simulink model "DA40_Flight_Model"  (R2023a)
settings: Solver=FixedStepAuto  StartTime=Start_Time  StopTime=End_Time  FixedStep=Time_Step  RelTol=1e-3
values from neighbouring files (symbols this model uses):
  BSFC_LUT = aircraft.BSFC_LUT    [NavigationProcessor.m]    (also in ReceiverPositions.m = obj.aircraft.BSFC_LUT; VectorTracking.m = load("DA40ENGINE.mat"))
  clkVar = formClkVariance(aircraft.clockType,1/aircraft.frequency)    [initializeSim.m]
  initP = blkdiag(diag([0.1 0.1 0.1]),diag([pi/90 pi/90 pi/90]),diag([1 1 1]),diag([pi/45 pi/45 pi/45]),clkVar)    [initializeSim.m]
  Q = blkdiag(diag(str2num(cell2mat(aircraft.noiseVariance))),clkVar)    [initializeSim.m]
  STGeometry = aircraft.STGeometry    [NavigationProcessor.m]    (also in ReceiverPositions.m = obj.aircraft.STGeometry; VectorTracking.m = load("DA40STGEOM.mat"))
  Vehicle = aircraft.Vehicle    [NavigationProcessor.m]    (also in ReceiverPositions.m = obj.aircraft.Vehicle; VectorTracking.m = load("DA40.mat"))
undefined symbols (not defined in the file or in its folder): day, initCN0, Initial_X, month, PowerFactor_LUT, Time_Step, unifrnd, variance, year
libraries: slpidlib x8, simulink_extras x3, aerolibwind2 x2, aerolibatmos2 x2, simulink x1
(part 2 of 2)

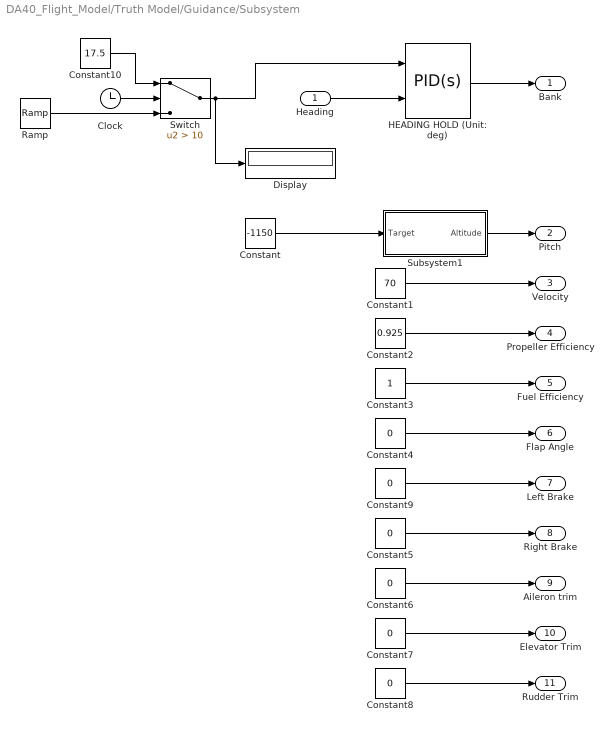
== system DA40_Flight_Model/Truth Model/Guidance/Subsystem ==
  Heading : Inport
  Clock : Clock
  Constant : Constant  Value=-1150
  Constant1 : Constant  Value=70
  Constant10 : Constant  Value=17.5
  Constant2 : Constant  Value=0.925
  Constant3 : Constant
  Constant{4..9} (6 alike) : Constant  Value=0
  Display : Display
  HEADING HOLD (Unit: deg) : slpidlib/PID Controller (2DOF)  Controller=PID  Form=Parallel  TimeDomain=Continuous-time  UseExternalTs=off  SampleTime=-1  IntegratorMethod=Forward Euler  FilterMethod=Forward Euler  ControllerParametersSource=internal  P=1  I=0.001  UseKiTs=off  D=0  N=100  UseFilter=on  b=1  c=0  TunerSelectOption=Transfer Function Based (PID Tuner App)  InitialConditionSource=internal  InitialConditionForIntegrator=0  InitialConditionForFilter=0  DifferentiatorICPrevScaledInput=0  ExternalReset=none  TrackingMode=off  Kt=1  LimitOutput=on  SatLimitsSource=internal  UpperSaturationLimit=30  LowerSaturationLimit=-30  LinearizeAsGain=on  AntiWindupMode=clamping  Kb=1  LimitIntegrator=off  UpperIntegratorSaturationLimit=inf  LowerIntegratorSaturationLimit=-inf  POutMin=[]  POutMax=[]  IOutMin=[]  IOutMax=[]  DOutMin=[]  DOutMax=[]  NOutMin=[]  NOutMax=[]  bOutMin=[]  bOutMax=[]  cOutMin=[]  cOutMax=[]  SumOutMin=[]  SumOutMax=[]  SaturationOutMin=[]  SaturationOutMax=[]  PParamMin=[]  PParamMax=[]  IParamMin=[]  IParamMax=[]  DParamMin=[]  DParamMax=[]  NParamMin=[]  NParamMax=[]  bParamMin=[]  bParamMax=[]  cParamMin=[]  cParamMax=[]  KbParamMin=[]  KbParamMax=[]  KtParamMin=[]  KtParamMax=[]  KbOutMin=[]  KbOutMax=[]  KtOutMin=[]  KtOutMax=[]  IntegratorOutMin=[]  IntegratorOutMax=[]  FilterOutMin=[]  FilterOutMax=[]  SumI1OutMin=[]  SumI1OutMax=[]  SumI2OutMin=[]  SumI2OutMax=[]  SumI3OutMin=[]  SumI3OutMax=[]  SumI4OutMin=[]  SumI4OutMax=[]  SumDOutMin=[]  SumDOutMax=[]  Sum1OutMin=[]  Sum1OutMax=[]  Sum2OutMin=[]  Sum2OutMax=[]  Sum3OutMin=[]  Sum3OutMax=[]  DifferentiatorOutMin=[]  DifferentiatorOutMax=[]  FilterDiffOutCoefMin=[]  FilterDiffOutCoefMax=[]  ReciprocalOutMin=[]  ReciprocalOutMax=[]  SumDenOutMin=[]  SumDenOutMax=[]  SumNumOutMin=[]  SumNumOutMax=[]  DivideOutMin=[]  DivideOutMax=[]  UdiffTsProdOutMin=[]  UdiffTsProdOutMax=[]  NTsProdOutMin=[]  NTsProdOutMax=[]  UintegralTsProdOutMin=[]  UintegralTsProdOutMax=[]  UngainTsProdOutMin=[]  UngainTsProdOutMax=[]  ClampingZeroOutDataTypeStr=Inherit: Inherit via back propagation  ClampingZeroOutMin=[]  ClampingZeroOutMax=[]  FilterDenConstantOutDataTypeStr=Inherit: Inherit via back propagation  FilterDenConstantOutMin=[]  FilterDenConstantOutMax=[]  PCopyOutDataTypeStr=Inherit: Inherit via back propagation  PCopyOutMin=[]  PCopyOutMax=[]  NCopyOutDataTypeStr=Inherit: Inherit via back propagation  NCopyOutMin=[]  NCopyOutMax=[]  IntegratorContinuousStateAttributes=''  IntegratorStateMustResolveToSignalObject=off  IntegratorRTWStateStorageClass=Auto  FilterContinuousStateAttributes=''  FilterStateMustResolveToSignalObject=off  FilterRTWStateStorageClass=Auto  ParallelPVariant=InternalParameters  IdealPVariant=Disabled  IVariant=InternalParameters  DVariant=InternalParameters  bVariant=InternalParameters  cVariant=InternalParameters  IntegratorVariant=Continuous  SatVariant=Enabled  AWVariant=ContClampingParallel  PCopyVariant=Disabled  TRVariant=Disabled  FdbkBlocksVariant=Forward  IdealPFdbkVariant=Disabled  SatFdbkVariant=Disabled  DerivativeFilterVariant=ContFilter  NVariant=InternalParameters  NCopyVariant=Disabled  FilterICVariant=InternalICsFilter  IntegratorICVariant=InternalICs  ExternalResetVariant=Disabled  TRSumVariant=Passthrough  SumFdbkVariant=Disabled  SumVariant=Sum_PID  TsampFilterVariant=InternalTs  TsampNgainVariant=Passthrough  TsampIntegralVariant=Disabled_SignalSpec  ExternalSaturationOutDataTypeStr=Inherit: Same as second input
  Ramp : simulink/Sources/Ramp  slope=2  start=1  InitialOutput=0  VectorParams1D=off
  Subsystem1 : Subsystem
  Switch : Switch  Criteria=u2 > Threshold  Threshold=10  SaturateOnIntegerOverflow=off  InputSameDT=off
  Bank : Outport
  Pitch : Outport  Port=2
  Velocity : Outport  Port=3
  Propeller Efficiency : Outport  Port=4
  Fuel Efficiency : Outport  Port=5
  Flap Angle : Outport  Port=6
  Left Brake : Outport  Port=7
  Right Brake : Outport  Port=8
  Aileron trim : Outport  Port=9
  Elevator Trim : Outport  Port=10
  Rudder Trim : Outport  Port=11
  wires:
  Subsystem1/1(Altitude) -> Pitch/1
  Constant1/1 -> Velocity/1
  Constant2/1 -> Propeller Efficiency/1
  Constant3/1 -> Fuel Efficiency/1
  Constant4/1 -> Flap Angle/1
  Constant9/1 -> Left Brake/1
  Constant5/1 -> Right Brake/1
  Constant6/1 -> Aileron trim/1
  Constant7/1 -> Elevator Trim/1
  Constant8/1 -> Rudder Trim/1
  HEADING HOLD (Unit: deg)/1 -> Bank/1
  Heading/1 -> HEADING HOLD (Unit: deg)/2
  Constant/1 -> Subsystem1/1(Target)
  Clock/1 -> Switch/2
  Ramp/1 -> Switch/3
  Constant10/1 -> Switch/1
  Switch/1 -> Display/1, HEADING HOLD (Unit: deg)/1

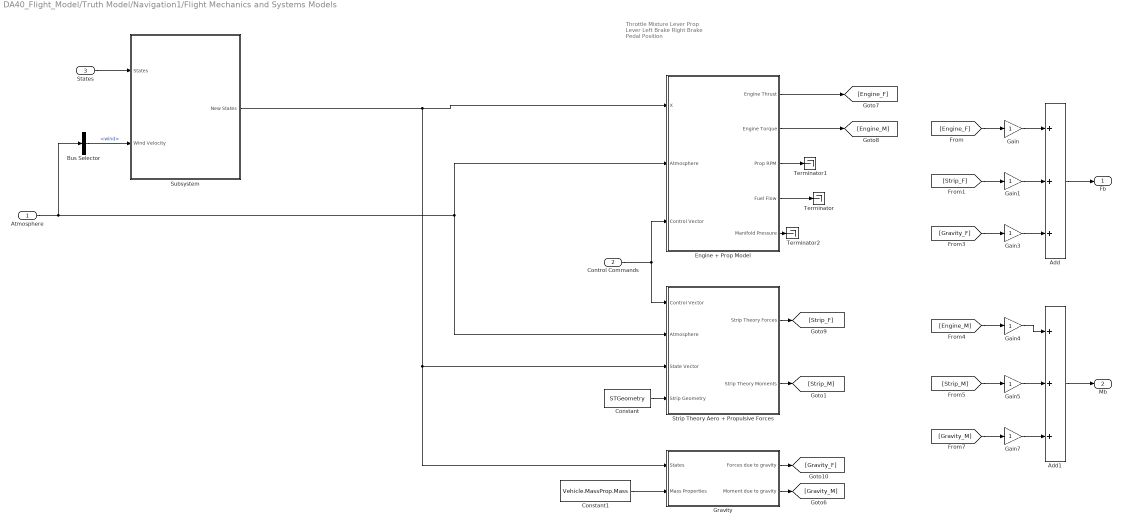
== system DA40_Flight_Model/Truth Model/Navigation1/Flight Mechanics and Systems Models ==
  note: Throttle
      | Mixture Lever
      | Prop Lever
      | Left Brake
      | Right Brake
      | Pedal Position
  Atmosphere : Inport
  Control Commands : Inport  Port=2
  States : Inport  Port=3
  Add : Sum  Inputs=+++
  Add1 : Sum  Inputs=+++
  Bus Selector : BusSelector  OutputSignals=wind
  Constant : Constant  Value=STGeometry
  Constant1 : Constant  Value=Vehicle.MassProp.Mass
  Engine + Prop Model : Subsystem
  Gain{,1,3..5,7} (6 alike) : Gain
  Gravity : Subsystem
  Strip Theory Aero + Propulsive Forces : Subsystem
  Subsystem : Subsystem
  Terminator : Terminator
  Terminator1 : Terminator
  Terminator2 : Terminator
  Fb : Outport
  Mb : Outport  Port=2
  wires:
  Constant1/1 -> Gravity/2(Mass Properties)
  Constant/1 -> Strip Theory Aero + Propulsive Forces/4(Strip Geometry)
  Engine + Prop Model/5(Manifold Pressure) -> Terminator2/1
  Engine + Prop Model/3(Prop RPM) -> Terminator1/1
  Add1/1 -> Mb/1
  Engine + Prop Model/2(Engine Torque) -> [Engine_M]
  Strip Theory Aero + Propulsive Forces/2(Strip Theory Moments) -> [Strip_M]
  Gravity/2(Moment due to gravity) -> [Gravity_M]
  Gravity/1(Forces due to gravity) -> [Gravity_F]
  Strip Theory Aero + Propulsive Forces/1(Strip Theory Forces) -> [Strip_F]
  Engine + Prop Model/1(Engine Thrust) -> [Engine_F]
  Add/1 -> Fb/1
  [Engine_F] -> Gain/1
  [Strip_F] -> Gain1/1
  [Gravity_F] -> Gain3/1
  [Engine_M] -> Gain4/1
  [Strip_M] -> Gain5/1
  [Gravity_M] -> Gain7/1
  Gain/1 -> Add/1
  Gain1/1 -> Add/2
  Gain3/1 -> Add/3
  Gain4/1 -> Add1/1
  Gain5/1 -> Add1/2
  Gain7/1 -> Add1/3
  Engine + Prop Model/4(Fuel Flow) -> Terminator/1
  Atmosphere/1 -> Bus Selector/1, Strip Theory Aero + Propulsive Forces/2(Atmosphere), Engine + Prop Model/2(Atmosphere)
  States/1 -> Subsystem/1(States)
  Control Commands/1 -> Strip Theory Aero + Propulsive Forces/1(Control Vector), Engine + Prop Model/3(Control Vector)
  Bus Selector/1 -> Subsystem/2(Wind Velocity)  "<wind>"
  Subsystem/1(New States) -> Gravity/1(States), Strip Theory Aero + Propulsive Forces/3(State Vector), Engine + Prop Model/1(X)

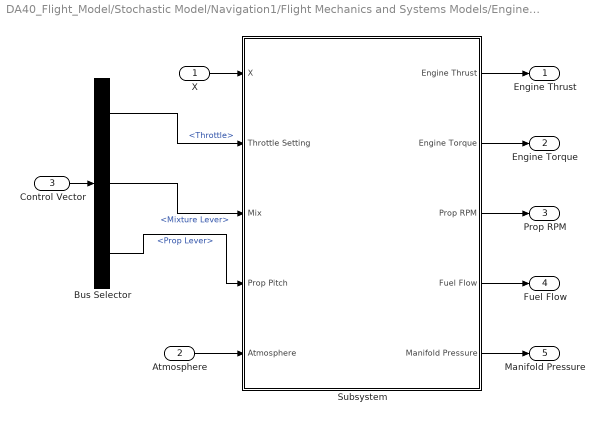
== system DA40_Flight_Model/Stochastic Model/Navigation1/Flight Mechanics and Systems Models/Engine + Prop Model ==
  X : Inport
  Atmosphere : Inport  Port=2
  Control Vector : Inport  Port=3
  Bus Selector : BusSelector  OutputSignals=Throttle,Mixture Lever,Prop Lever
  Subsystem : Subsystem
  Engine Thrust : Outport
  Engine Torque : Outport  Port=2
  Prop RPM : Outport  Port=3  PortDimensions=1
  Fuel Flow : Outport  Port=4  PortDimensions=1
  Manifold Pressure : Outport  Port=5  PortDimensions=1
  wires:
  X/1 -> Subsystem/1(X)
  Subsystem/3(Prop RPM) -> Prop RPM/1
  Subsystem/4(Fuel Flow) -> Fuel Flow/1
  Subsystem/5(Manifold Pressure) -> Manifold Pressure/1
  Control Vector/1 -> Bus Selector/1
  Bus Selector/1 -> Subsystem/2(Throttle Setting)  "<Throttle>"
  Bus Selector/2 -> Subsystem/3(Mix)  "<Mixture Lever>"
  Bus Selector/3 -> Subsystem/4(Prop Pitch)  "<Prop Lever>"
  Atmosphere/1 -> Subsystem/5(Atmosphere)
  Subsystem/2(Engine Torque) -> Engine Torque/1
  Subsystem/1(Engine Thrust) -> Engine Thrust/1

== system DA40_Flight_Model/Stochastic Model/Navigation1/Flight Mechanics and Systems Models/Gravity ==
  States : Inport
  Mass Properties : Inport  Port=2
  Constant : Constant  Value=Vehicle.MassProp.r_cg
  MATLAB Function : MATLAB Function  TreatAsAtomicUnit=on
  Forces due to gravity : Outport
  Moment due to gravity : Outport  Port=2
  wires:
  MATLAB Function/1(F_grav_b) -> Forces due to gravity/1
  States/1 -> MATLAB Function/1(X)
  Mass Properties/1 -> MATLAB Function/2(Mass_Properties)
  MATLAB Function/2(M_grav_b) -> Moment due to gravity/1
  Constant/1 -> MATLAB Function/3(CG)

== system DA40_Flight_Model/Stochastic Model/Navigation1/Flight Mechanics and Systems Models/Strip Theory Aero + Propulsive Forces ==
  Control Vector : Inport
  Atmosphere : Inport  Port=2
  State Vector : Inport  Port=3
  Strip Geometry : Inport  Port=4
  Strip_Theory_Modeling : MATLAB Function  TreatAsAtomicUnit=on
  Strip Theory Forces : Outport
  Strip Theory Moments : Outport  Port=2
  wires:
  Atmosphere/1 -> Strip_Theory_Modeling/1(atmos)
  Strip Geometry/1 -> Strip_Theory_Modeling/4(stripGeom)
  Control Vector/1 -> Strip_Theory_Modeling/3(U)
  State Vector/1 -> Strip_Theory_Modeling/2(X)
  Strip_Theory_Modeling/1(Strip_Theory_Forces) -> Strip Theory Forces/1
  Strip_Theory_Modeling/2(Strip_Theory_Moments) -> Strip Theory Moments/1

== system DA40_Flight_Model/Stochastic Model/Navigation1/Flight Mechanics and Systems Models/Subsystem ==
  States : Inport
  Wind Velocity : Inport  Port=2
  Add : Sum  Inputs=-+
  Demux : Demux  Outputs=14
  Demux1 : Demux  Outputs=3
  Mux : Mux  Inputs=14
  Mux1 : Mux  Inputs=3
  New States : Outport
  wires:
  States/1 -> Demux/1
  Mux/1 -> New States/1
  Demux/12 -> Mux/12
  Demux/11 -> Mux/11
  Demux/10 -> Mux/10
  Demux/9 -> Mux/9
  Demux/8 -> Mux/8
  Demux/7 -> Mux/7
  Demux/6 -> Mux/6
  Demux/5 -> Mux/5
  Demux/4 -> Mux/4
  Demux/1 -> Mux1/1
  Demux/2 -> Mux1/2
  Demux/3 -> Mux1/3
  Wind Velocity/1 -> Add/1
  Mux1/1 -> Add/2
  Demux1/1 -> Mux/1
  Demux1/2 -> Mux/2
  Demux1/3 -> Mux/3
  Add/1 -> Demux1/1
  Demux/13 -> Mux/13
  Demux/14 -> Mux/14

== system DA40_Flight_Model/Truth Model/Guidance/Subsystem/Subsystem1 ==
  Target : Inport
  Gain : Gain  Gain=-1
  Altitude : Outport
  wires:
  Target/1 -> Gain/1
  Gain/1 -> Altitude/1

== system DA40_Flight_Model/Truth Model/Navigation1/Flight Mechanics and Systems Models/Engine + Prop Model ==
  X : Inport
  Atmosphere : Inport  Port=2
  Control Vector : Inport  Port=3
  Bus Selector : BusSelector  OutputSignals=Throttle,Mixture Lever,Prop Lever
  Subsystem : Subsystem
  Engine Thrust : Outport
  Engine Torque : Outport  Port=2
  Prop RPM : Outport  Port=3  PortDimensions=1
  Fuel Flow : Outport  Port=4  PortDimensions=1
  Manifold Pressure : Outport  Port=5  PortDimensions=1
  wires:
  X/1 -> Subsystem/1(X)
  Subsystem/3(Prop RPM) -> Prop RPM/1
  Subsystem/4(Fuel Flow) -> Fuel Flow/1
  Subsystem/5(Manifold Pressure) -> Manifold Pressure/1
  Control Vector/1 -> Bus Selector/1
  Bus Selector/1 -> Subsystem/2(Throttle Setting)  "<Throttle>"
  Bus Selector/2 -> Subsystem/3(Mix)  "<Mixture Lever>"
  Bus Selector/3 -> Subsystem/4(Prop Pitch)  "<Prop Lever>"
  Atmosphere/1 -> Subsystem/5(Atmosphere)
  Subsystem/2(Engine Torque) -> Engine Torque/1
  Subsystem/1(Engine Thrust) -> Engine Thrust/1

== system DA40_Flight_Model/Truth Model/Navigation1/Flight Mechanics and Systems Models/Gravity ==
  States : Inport
  Mass Properties : Inport  Port=2
  Constant : Constant  Value=Vehicle.MassProp.r_cg
  MATLAB Function : MATLAB Function  TreatAsAtomicUnit=on
  Forces due to gravity : Outport
  Moment due to gravity : Outport  Port=2
  wires:
  MATLAB Function/1(F_grav_b) -> Forces due to gravity/1
  States/1 -> MATLAB Function/1(X)
  Mass Properties/1 -> MATLAB Function/2(Mass_Properties)
  MATLAB Function/2(M_grav_b) -> Moment due to gravity/1
  Constant/1 -> MATLAB Function/3(CG)

== system DA40_Flight_Model/Truth Model/Navigation1/Flight Mechanics and Systems Models/Strip Theory Aero + Propulsive Forces ==
  Control Vector : Inport
  Atmosphere : Inport  Port=2
  State Vector : Inport  Port=3
  Strip Geometry : Inport  Port=4
  Strip_Theory_Modeling : MATLAB Function  TreatAsAtomicUnit=on
  Strip Theory Forces : Outport
  Strip Theory Moments : Outport  Port=2
  wires:
  Atmosphere/1 -> Strip_Theory_Modeling/1(atmos)
  Strip Geometry/1 -> Strip_Theory_Modeling/4(stripGeom)
  Control Vector/1 -> Strip_Theory_Modeling/3(U)
  State Vector/1 -> Strip_Theory_Modeling/2(X)
  Strip_Theory_Modeling/1(Strip_Theory_Forces) -> Strip Theory Forces/1
  Strip_Theory_Modeling/2(Strip_Theory_Moments) -> Strip Theory Moments/1

== system DA40_Flight_Model/Truth Model/Navigation1/Flight Mechanics and Systems Models/Subsystem ==
  States : Inport
  Wind Velocity : Inport  Port=2
  Add : Sum  Inputs=-+
  Demux : Demux  Outputs=14
  Demux1 : Demux  Outputs=3
  Mux : Mux  Inputs=14
  Mux1 : Mux  Inputs=3
  New States : Outport
  wires:
  States/1 -> Demux/1
  Mux/1 -> New States/1
  Demux/12 -> Mux/12
  Demux/11 -> Mux/11
  Demux/10 -> Mux/10
  Demux/9 -> Mux/9
  Demux/8 -> Mux/8
  Demux/7 -> Mux/7
  Demux/6 -> Mux/6
  Demux/5 -> Mux/5
  Demux/4 -> Mux/4
  Demux/1 -> Mux1/1
  Demux/2 -> Mux1/2
  Demux/3 -> Mux1/3
  Wind Velocity/1 -> Add/1
  Mux1/1 -> Add/2
  Demux1/1 -> Mux/1
  Demux1/2 -> Mux/2
  Demux1/3 -> Mux/3
  Add/1 -> Demux1/1
  Demux/13 -> Mux/13
  Demux/14 -> Mux/14

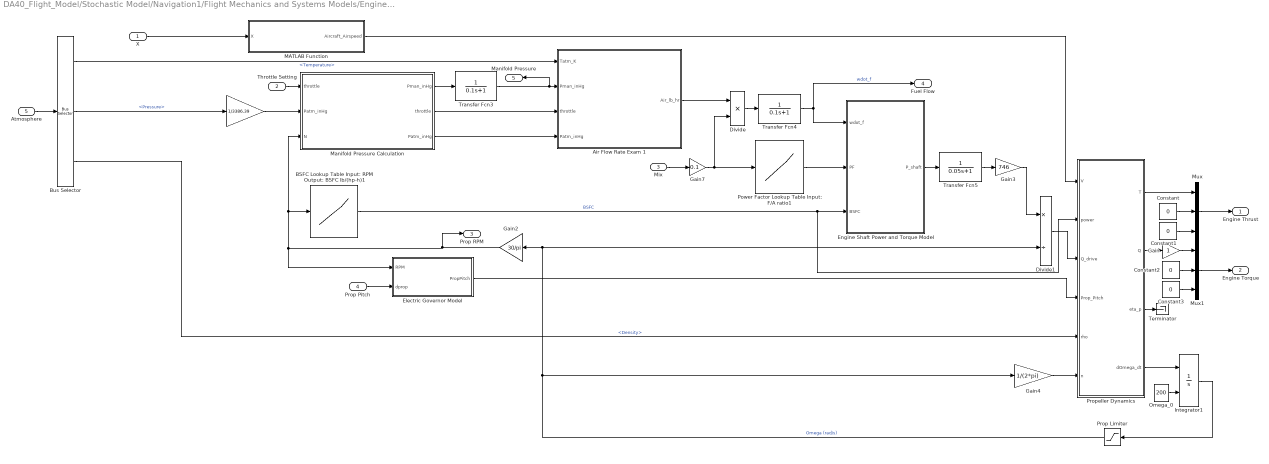
== system DA40_Flight_Model/Stochastic Model/Navigation1/Flight Mechanics and Systems Models/Engine + Prop Model/Subsystem ==
  X : Inport
  Throttle Setting : Inport  Port=2
  Mix : Inport  Port=3
  Prop Pitch : Inport  Port=4
  Atmosphere : Inport  Port=5
  " " : Gain  Gain=1/3386.39
  Air Flow Rate Exam 1 : MATLAB Function  TreatAsAtomicUnit=on
  BSFC Lookup Table Input: RPM Output: BSFC lb/(hp-h)1 : Lookup_n-D  NumberOfTableDimensions=1  BreakpointsForDimension1=BSFC_LUT(1,:)  Table=BSFC_LUT(2,:)  ExtrapMethod=Clip  UseLastTableValue=on  InternalRulePriority=Speed  RndMeth=Simplest
  Bus Selector : BusSelector  OutputSignals=Temperature,Pressure,Density
  Constant{,1..3} (4 alike) : Constant  Value=0
  Divide : Product  Inputs=**
  Divide1 : Product  Inputs=*/
  Electric Governor Model : Subsystem
  Engine Shaft Power and Torque Model : MATLAB Function  TreatAsAtomicUnit=on
  Gain : Gain
  Gain2 : Gain  Gain=30/pi
  Gain3 : Gain  Gain=746
  Gain4 : Gain  Gain=1/(2*pi)
  Gain7 : Gain  Gain=0.1
  Integrator1 : Integrator  InitialConditionSource=external
  MATLAB Function : MATLAB Function  TreatAsAtomicUnit=on
  Manifold Pressure Calculation : MATLAB Function  TreatAsAtomicUnit=on
  Mux : Mux  Inputs=3
  Mux1 : Mux  Inputs=3
  Omega_0 : Constant  Value=200
  Power Factor Lookup Table Input: F/A ratio1 : Lookup_n-D  NumberOfTableDimensions=1  BreakpointsForDimension1=PowerFactor_LUT(1,:)  Table=PowerFactor_LUT(2,:)  ExtrapMethod=Clip  UseLastTableValue=on  InternalRulePriority=Speed  RndMeth=Simplest
  Prop Limiter : Saturate  UpperLimit=320  LowerLimit=0
  Propeller Dynamics : MATLAB Function  TreatAsAtomicUnit=on
  Terminator : Terminator
  Transfer Fcn3 : TransferFcn  Denominator=[0.1 1]
  Transfer Fcn4 : TransferFcn  Denominator=[0.1 1]
  Transfer Fcn5 : TransferFcn  Denominator=[0.05 1]
  Engine Thrust : Outport
  Engine Torque : Outport  Port=2
  Prop RPM : Outport  Port=3  PortDimensions=1
  Fuel Flow : Outport  Port=4  PortDimensions=1
  Manifold Pressure : Outport  Port=5  PortDimensions=1
  wires:
  Transfer Fcn4/1 -> Engine Shaft Power and Torque Model/1(wdot_f), Fuel Flow/1  "wdot_f"
  Constant2/1 -> Mux1/2
  Propeller Dynamics/4(dOmega_dt) -> Integrator1/1
  Mux/1 -> Engine Thrust/1
  Gain2/1 -> Prop RPM/1, Electric Governor Model/1(RPM), BSFC Lookup Table Input: RPM Output: BSFC lb/(hp-h)1/1, Manifold Pressure Calculation/3(N)
  Electric Governor Model/1(PropPitch) -> Propeller Dynamics/4(Prop_Pitch)
  Divide/1 -> Transfer Fcn4/1
  Constant/1 -> Mux/2
  Gain4/1 -> Propeller Dynamics/6(n)
  Mix/1 -> Gain7/1
  Bus Selector/3 -> Propeller Dynamics/5(rho)  "<Density>"
  Manifold Pressure Calculation/3(Patm_inHg) -> Air Flow Rate Exam 1/4(Patm_inHg)
  BSFC Lookup Table Input: RPM Output: BSFC lb/(hp-h)1/1 -> Propeller Dynamics/2(power), Engine Shaft Power and Torque Model/3(BSFC)  "BSFC"
  Manifold Pressure Calculation/2(throttle) -> Air Flow Rate Exam 1/3(throttle)
  Prop Limiter/1 -> Divide1/2, Gain2/1, Gain4/1  "Omega (rad/s)"
  Propeller Dynamics/1(T) -> Mux/1
  Engine Shaft Power and Torque Model/1(P_shaft) -> Transfer Fcn5/1
  Omega_0/1 -> Integrator1/2
  Constant3/1 -> Mux1/3
  Transfer Fcn3/1 -> Manifold Pressure/1, Air Flow Rate Exam 1/2(Pman_inHg)
  Power Factor Lookup Table Input: F/A ratio1/1 -> Engine Shaft Power and Torque Model/2(PF)
  X/1 -> MATLAB Function/1(X)
  Gain3/1 -> Divide1/1
  Prop Pitch/1 -> Electric Governor Model/2(dprop)
  Transfer Fcn5/1 -> Gain3/1
  Propeller Dynamics/2(Q) -> Gain/1
  Mux1/1 -> Engine Torque/1
  Gain/1 -> Mux1/1
  Divide1/1 -> Propeller Dynamics/3(Q_drive)
  Manifold Pressure Calculation/1(Pman_inHg) -> Transfer Fcn3/1
  Gain7/1 -> Power Factor Lookup Table Input: F/A ratio1/1, Divide/2
  MATLAB Function/1(Aircraft_Airspeed) -> Propeller Dynamics/1(V)
  Throttle Setting/1 -> Manifold Pressure Calculation/1("throttle ")
  " "/1 -> Manifold Pressure Calculation/2("Patm_inHg ")
  Constant1/1 -> Mux/3
  Atmosphere/1 -> Bus Selector/1
  Bus Selector/1 -> Air Flow Rate Exam 1/1(Tatm_K)  "<Temperature>"
  Bus Selector/2 -> " "/1  "<Pressure>"
  Air Flow Rate Exam 1/1(Air_lb_hr) -> Divide/1
  Integrator1/1 -> Prop Limiter/1
  Propeller Dynamics/3(eta_p) -> Terminator/1

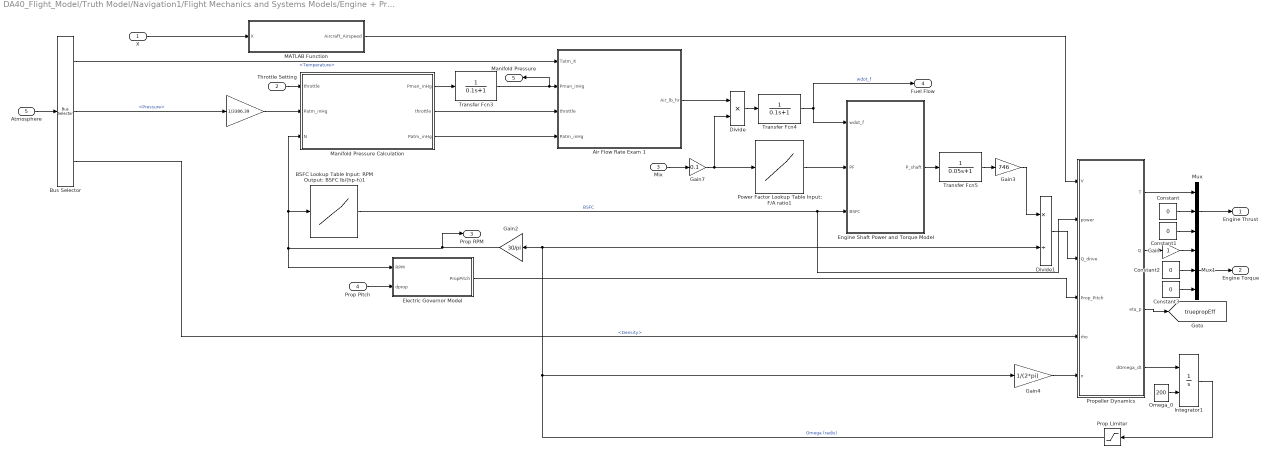
== system DA40_Flight_Model/Truth Model/Navigation1/Flight Mechanics and Systems Models/Engine + Prop Model/Subsystem ==
  X : Inport
  Throttle Setting : Inport  Port=2
  Mix : Inport  Port=3
  Prop Pitch : Inport  Port=4
  Atmosphere : Inport  Port=5
  " " : Gain  Gain=1/3386.39
  Air Flow Rate Exam 1 : MATLAB Function  TreatAsAtomicUnit=on
  BSFC Lookup Table Input: RPM Output: BSFC lb/(hp-h)1 : Lookup_n-D  NumberOfTableDimensions=1  BreakpointsForDimension1=BSFC_LUT(1,:)  Table=BSFC_LUT(2,:)  ExtrapMethod=Clip  UseLastTableValue=on  InternalRulePriority=Speed  RndMeth=Simplest
  Bus Selector : BusSelector  OutputSignals=Temperature,Pressure,Density
  Constant{,1..3} (4 alike) : Constant  Value=0
  Divide : Product  Inputs=**
  Divide1 : Product  Inputs=*/
  Electric Governor Model : Subsystem
  Engine Shaft Power and Torque Model : MATLAB Function  TreatAsAtomicUnit=on
  Gain : Gain
  Gain2 : Gain  Gain=30/pi
  Gain3 : Gain  Gain=746
  Gain4 : Gain  Gain=1/(2*pi)
  Gain7 : Gain  Gain=0.1
  Integrator1 : Integrator  InitialConditionSource=external
  MATLAB Function : MATLAB Function  TreatAsAtomicUnit=on
  Manifold Pressure Calculation : MATLAB Function  TreatAsAtomicUnit=on
  Mux : Mux  Inputs=3
  Mux1 : Mux  Inputs=3
  Omega_0 : Constant  Value=200
  Power Factor Lookup Table Input: F/A ratio1 : Lookup_n-D  NumberOfTableDimensions=1  BreakpointsForDimension1=PowerFactor_LUT(1,:)  Table=PowerFactor_LUT(2,:)  ExtrapMethod=Clip  UseLastTableValue=on  InternalRulePriority=Speed  RndMeth=Simplest
  Prop Limiter : Saturate  UpperLimit=320  LowerLimit=0
  Propeller Dynamics : MATLAB Function  TreatAsAtomicUnit=on
  Transfer Fcn3 : TransferFcn  Denominator=[0.1 1]
  Transfer Fcn4 : TransferFcn  Denominator=[0.1 1]
  Transfer Fcn5 : TransferFcn  Denominator=[0.05 1]
  Engine Thrust : Outport
  Engine Torque : Outport  Port=2
  Prop RPM : Outport  Port=3  PortDimensions=1
  Fuel Flow : Outport  Port=4  PortDimensions=1
  Manifold Pressure : Outport  Port=5  PortDimensions=1
  tag scope: truepropEff=global
  wires:
  Transfer Fcn4/1 -> Engine Shaft Power and Torque Model/1(wdot_f), Fuel Flow/1  "wdot_f"
  Constant2/1 -> Mux1/2
  Propeller Dynamics/4(dOmega_dt) -> Integrator1/1
  Mux/1 -> Engine Thrust/1
  Gain2/1 -> Prop RPM/1, Electric Governor Model/1(RPM), BSFC Lookup Table Input: RPM Output: BSFC lb/(hp-h)1/1, Manifold Pressure Calculation/3(N)
  Electric Governor Model/1(PropPitch) -> Propeller Dynamics/4(Prop_Pitch)
  Divide/1 -> Transfer Fcn4/1
  Propeller Dynamics/3(eta_p) -> [truepropEff]
  Constant/1 -> Mux/2
  Gain4/1 -> Propeller Dynamics/6(n)
  Mix/1 -> Gain7/1
  Bus Selector/3 -> Propeller Dynamics/5(rho)  "<Density>"
  Manifold Pressure Calculation/3(Patm_inHg) -> Air Flow Rate Exam 1/4(Patm_inHg)
  BSFC Lookup Table Input: RPM Output: BSFC lb/(hp-h)1/1 -> Propeller Dynamics/2(power), Engine Shaft Power and Torque Model/3(BSFC)  "BSFC"
  Manifold Pressure Calculation/2(throttle) -> Air Flow Rate Exam 1/3(throttle)
  Prop Limiter/1 -> Divide1/2, Gain2/1, Gain4/1  "Omega (rad/s)"
  Propeller Dynamics/1(T) -> Mux/1
  Engine Shaft Power and Torque Model/1(P_shaft) -> Transfer Fcn5/1
  Omega_0/1 -> Integrator1/2
  Constant3/1 -> Mux1/3
  Transfer Fcn3/1 -> Manifold Pressure/1, Air Flow Rate Exam 1/2(Pman_inHg)
  Power Factor Lookup Table Input: F/A ratio1/1 -> Engine Shaft Power and Torque Model/2(PF)
  X/1 -> MATLAB Function/1(X)
  Gain3/1 -> Divide1/1
  Prop Pitch/1 -> Electric Governor Model/2(dprop)
  Transfer Fcn5/1 -> Gain3/1
  Propeller Dynamics/2(Q) -> Gain/1
  Mux1/1 -> Engine Torque/1
  Gain/1 -> Mux1/1
  Divide1/1 -> Propeller Dynamics/3(Q_drive)
  Manifold Pressure Calculation/1(Pman_inHg) -> Transfer Fcn3/1
  Gain7/1 -> Power Factor Lookup Table Input: F/A ratio1/1, Divide/2
  MATLAB Function/1(Aircraft_Airspeed) -> Propeller Dynamics/1(V)
  Throttle Setting/1 -> Manifold Pressure Calculation/1("throttle ")
  " "/1 -> Manifold Pressure Calculation/2("Patm_inHg ")
  Constant1/1 -> Mux/3
  Atmosphere/1 -> Bus Selector/1
  Bus Selector/1 -> Air Flow Rate Exam 1/1(Tatm_K)  "<Temperature>"
  Bus Selector/2 -> " "/1  "<Pressure>"
  Air Flow Rate Exam 1/1(Air_lb_hr) -> Divide/1
  Integrator1/1 -> Prop Limiter/1

== system DA40_Flight_Model/Stochastic Model/Navigation1/Flight Mechanics and Systems Models/Engine + Prop Model/Subsystem/Electric Governor Model ==
  RPM : Inport
  dprop : Inport  Port=2
  Constant : Constant  Value=0
  DESIRED RPM : MATLABFcn  MATLABFcn=800 + 2000 * u
  Initial Blade Pitch : Constant  Value=5
  PID Controller (2DOF) : slpidlib/PID Controller (2DOF)  Controller=PID  Form=Parallel  TimeDomain=Continuous-time  UseExternalTs=off  SampleTime=-1  IntegratorMethod=Forward Euler  FilterMethod=Forward Euler  ControllerParametersSource=internal  P=-.08  I=-0.01  UseKiTs=off  D=0  N=100  UseFilter=on  b=1  c=0  TunerSelectOption=Transfer Function Based (PID Tuner App)  InitialConditionSource=external  InitialConditionForIntegrator=0  InitialConditionForFilter=0  DifferentiatorICPrevScaledInput=0  ExternalReset=none  TrackingMode=off  Kt=1  LimitOutput=on  SatLimitsSource=internal  UpperSaturationLimit=26  LowerSaturationLimit=10  LinearizeAsGain=on  AntiWindupMode=clamping  Kb=1  LimitIntegrator=off  UpperIntegratorSaturationLimit=inf  LowerIntegratorSaturationLimit=-inf  POutMin=[]  POutMax=[]  IOutMin=[]  IOutMax=[]  DOutMin=[]  DOutMax=[]  NOutMin=[]  NOutMax=[]  bOutMin=[]  bOutMax=[]  cOutMin=[]  cOutMax=[]  SumOutMin=[]  SumOutMax=[]  SaturationOutMin=[]  SaturationOutMax=[]  PParamMin=[]  PParamMax=[]  IParamMin=[]  IParamMax=[]  DParamMin=[]  DParamMax=[]  NParamMin=[]  NParamMax=[]  bParamMin=[]  bParamMax=[]  cParamMin=[]  cParamMax=[]  KbParamMin=[]  KbParamMax=[]  KtParamMin=[]  KtParamMax=[]  KbOutMin=[]  KbOutMax=[]  KtOutMin=[]  KtOutMax=[]  IntegratorOutMin=[]  IntegratorOutMax=[]  FilterOutMin=[]  FilterOutMax=[]  SumI1OutMin=[]  SumI1OutMax=[]  SumI2OutMin=[]  SumI2OutMax=[]  SumI3OutMin=[]  SumI3OutMax=[]  SumI4OutMin=[]  SumI4OutMax=[]  SumDOutMin=[]  SumDOutMax=[]  Sum1OutMin=[]  Sum1OutMax=[]  Sum2OutMin=[]  Sum2OutMax=[]  Sum3OutMin=[]  Sum3OutMax=[]  DifferentiatorOutMin=[]  DifferentiatorOutMax=[]  FilterDiffOutCoefMin=[]  FilterDiffOutCoefMax=[]  ReciprocalOutMin=[]  ReciprocalOutMax=[]  SumDenOutMin=[]  SumDenOutMax=[]  SumNumOutMin=[]  SumNumOutMax=[]  DivideOutMin=[]  DivideOutMax=[]  UdiffTsProdOutMin=[]  UdiffTsProdOutMax=[]  NTsProdOutMin=[]  NTsProdOutMax=[]  UintegralTsProdOutMin=[]  UintegralTsProdOutMax=[]  UngainTsProdOutMin=[]  UngainTsProdOutMax=[]  ClampingZeroOutDataTypeStr=Inherit: Inherit via back propagation  ClampingZeroOutMin=[]  ClampingZeroOutMax=[]  FilterDenConstantOutDataTypeStr=Inherit: Inherit via back propagation  FilterDenConstantOutMin=[]  FilterDenConstantOutMax=[]  PCopyOutDataTypeStr=Inherit: Inherit via back propagation  PCopyOutMin=[]  PCopyOutMax=[]  NCopyOutDataTypeStr=Inherit: Inherit via back propagation  NCopyOutMin=[]  NCopyOutMax=[]  IntegratorContinuousStateAttributes=''  IntegratorStateMustResolveToSignalObject=off  IntegratorRTWStateStorageClass=Auto  FilterContinuousStateAttributes=''  FilterStateMustResolveToSignalObject=off  FilterRTWStateStorageClass=Auto  ParallelPVariant=InternalParameters  IdealPVariant=Disabled  IVariant=InternalParameters  DVariant=InternalParameters  bVariant=InternalParameters  cVariant=InternalParameters  IntegratorVariant=Continuous  SatVariant=Enabled  AWVariant=ContClampingParallel  PCopyVariant=Disabled  TRVariant=Disabled  FdbkBlocksVariant=Forward  IdealPFdbkVariant=Disabled  SatFdbkVariant=Disabled  DerivativeFilterVariant=ContFilter  NVariant=InternalParameters  NCopyVariant=Disabled  FilterICVariant=ExternalICs  IntegratorICVariant=ExternalICs  ExternalResetVariant=Disabled  TRSumVariant=Passthrough  SumFdbkVariant=Disabled  SumVariant=Sum_PID  TsampFilterVariant=InternalTs  TsampNgainVariant=Passthrough  TsampIntegralVariant=Disabled_SignalSpec  ExternalSaturationOutDataTypeStr=Inherit: Same as second input
  Saturation : Saturate  UpperLimit=2650  LowerLimit=800
  PropPitch : Outport
  wires:
  dprop/1 -> DESIRED RPM/1
  PID Controller (2DOF)/1 -> PropPitch/1
  Constant/1 -> PID Controller (2DOF)/4
  Initial Blade Pitch/1 -> PID Controller (2DOF)/3
  DESIRED RPM/1 -> Saturation/1
  RPM/1 -> PID Controller (2DOF)/2
  Saturation/1 -> PID Controller (2DOF)/1

== system DA40_Flight_Model/Truth Model/Navigation1/Flight Mechanics and Systems Models/Engine + Prop Model/Subsystem/Electric Governor Model ==
  RPM : Inport
  dprop : Inport  Port=2
  Constant : Constant  Value=0
  DESIRED RPM : MATLABFcn  MATLABFcn=800 + 2000 * u
  Initial Blade Pitch : Constant  Value=5
  PID Controller (2DOF) : slpidlib/PID Controller (2DOF)  Controller=PID  Form=Parallel  TimeDomain=Continuous-time  UseExternalTs=off  SampleTime=-1  IntegratorMethod=Forward Euler  FilterMethod=Forward Euler  ControllerParametersSource=internal  P=-.08  I=-0.01  UseKiTs=off  D=0  N=100  UseFilter=on  b=1  c=0  TunerSelectOption=Transfer Function Based (PID Tuner App)  InitialConditionSource=external  InitialConditionForIntegrator=0  InitialConditionForFilter=0  DifferentiatorICPrevScaledInput=0  ExternalReset=none  TrackingMode=off  Kt=1  LimitOutput=on  SatLimitsSource=internal  UpperSaturationLimit=26  LowerSaturationLimit=10  LinearizeAsGain=on  AntiWindupMode=clamping  Kb=1  LimitIntegrator=off  UpperIntegratorSaturationLimit=inf  LowerIntegratorSaturationLimit=-inf  POutMin=[]  POutMax=[]  IOutMin=[]  IOutMax=[]  DOutMin=[]  DOutMax=[]  NOutMin=[]  NOutMax=[]  bOutMin=[]  bOutMax=[]  cOutMin=[]  cOutMax=[]  SumOutMin=[]  SumOutMax=[]  SaturationOutMin=[]  SaturationOutMax=[]  PParamMin=[]  PParamMax=[]  IParamMin=[]  IParamMax=[]  DParamMin=[]  DParamMax=[]  NParamMin=[]  NParamMax=[]  bParamMin=[]  bParamMax=[]  cParamMin=[]  cParamMax=[]  KbParamMin=[]  KbParamMax=[]  KtParamMin=[]  KtParamMax=[]  KbOutMin=[]  KbOutMax=[]  KtOutMin=[]  KtOutMax=[]  IntegratorOutMin=[]  IntegratorOutMax=[]  FilterOutMin=[]  FilterOutMax=[]  SumI1OutMin=[]  SumI1OutMax=[]  SumI2OutMin=[]  SumI2OutMax=[]  SumI3OutMin=[]  SumI3OutMax=[]  SumI4OutMin=[]  SumI4OutMax=[]  SumDOutMin=[]  SumDOutMax=[]  Sum1OutMin=[]  Sum1OutMax=[]  Sum2OutMin=[]  Sum2OutMax=[]  Sum3OutMin=[]  Sum3OutMax=[]  DifferentiatorOutMin=[]  DifferentiatorOutMax=[]  FilterDiffOutCoefMin=[]  FilterDiffOutCoefMax=[]  ReciprocalOutMin=[]  ReciprocalOutMax=[]  SumDenOutMin=[]  SumDenOutMax=[]  SumNumOutMin=[]  SumNumOutMax=[]  DivideOutMin=[]  DivideOutMax=[]  UdiffTsProdOutMin=[]  UdiffTsProdOutMax=[]  NTsProdOutMin=[]  NTsProdOutMax=[]  UintegralTsProdOutMin=[]  UintegralTsProdOutMax=[]  UngainTsProdOutMin=[]  UngainTsProdOutMax=[]  ClampingZeroOutDataTypeStr=Inherit: Inherit via back propagation  ClampingZeroOutMin=[]  ClampingZeroOutMax=[]  FilterDenConstantOutDataTypeStr=Inherit: Inherit via back propagation  FilterDenConstantOutMin=[]  FilterDenConstantOutMax=[]  PCopyOutDataTypeStr=Inherit: Inherit via back propagation  PCopyOutMin=[]  PCopyOutMax=[]  NCopyOutDataTypeStr=Inherit: Inherit via back propagation  NCopyOutMin=[]  NCopyOutMax=[]  IntegratorContinuousStateAttributes=''  IntegratorStateMustResolveToSignalObject=off  IntegratorRTWStateStorageClass=Auto  FilterContinuousStateAttributes=''  FilterStateMustResolveToSignalObject=off  FilterRTWStateStorageClass=Auto  ParallelPVariant=InternalParameters  IdealPVariant=Disabled  IVariant=InternalParameters  DVariant=InternalParameters  bVariant=InternalParameters  cVariant=InternalParameters  IntegratorVariant=Continuous  SatVariant=Enabled  AWVariant=ContClampingParallel  PCopyVariant=Disabled  TRVariant=Disabled  FdbkBlocksVariant=Forward  IdealPFdbkVariant=Disabled  SatFdbkVariant=Disabled  DerivativeFilterVariant=ContFilter  NVariant=InternalParameters  NCopyVariant=Disabled  FilterICVariant=ExternalICs  IntegratorICVariant=ExternalICs  ExternalResetVariant=Disabled  TRSumVariant=Passthrough  SumFdbkVariant=Disabled  SumVariant=Sum_PID  TsampFilterVariant=InternalTs  TsampNgainVariant=Passthrough  TsampIntegralVariant=Disabled_SignalSpec  ExternalSaturationOutDataTypeStr=Inherit: Same as second input
  Saturation : Saturate  UpperLimit=2650  LowerLimit=800
  PropPitch : Outport
  wires:
  dprop/1 -> DESIRED RPM/1
  PID Controller (2DOF)/1 -> PropPitch/1
  Constant/1 -> PID Controller (2DOF)/4
  Initial Blade Pitch/1 -> PID Controller (2DOF)/3
  DESIRED RPM/1 -> Saturation/1
  RPM/1 -> PID Controller (2DOF)/2
  Saturation/1 -> PID Controller (2DOF)/1

== matlab function DA40_Flight_Model/Stochastic Model/Environment/MATLAB Function7 ==
  data: RotAngles input; DCM output; RotSequence input
function DCM = MyDCMFunction(RotAngles,RotSequence)
n = length(RotSequence);
Matrix = zeros(3,3,3);
for i = 1:n
    k = RotSequence(i);
    switch k
        case 1
            Matrix(:,:,i) = [1 0 0;0 cosd(RotAngles(i)) -sind(RotAngles(i));0 sind(RotAngles(i)) cosd(RotAngles(i))];
        case 2
            Matrix(:,:,i) = [cosd(RotAngles(i)) 0 sind(RotAngles(i));0 1 0;-sind(RotAngles(i)) 0 cosd(RotAngles(i))];
        case 3
            Matrix(:,:,i) = [cosd(RotAngles(i)) -sind(RotAngles(i)) 0;sind(RotAngles(i)) cosd(RotAngles(i)) 0;0 0 1];
    end
end
p = 1;
while p < n
    Matrix(:,:,p+1) = Matrix(:,:,p) * Matrix(:,:,p+1);
    p = p + 1;
end
DCM = Matrix(:,:,p);
end

== matlab function DA40_Flight_Model/Stochastic Model/Navigation1/Flight Mechanics and Systems Models/Engine + Prop Model/Subsystem/Air Flow Rate Exam 1 ==
  data: Tatm_K input; Pman_inHg input; throttle input; Patm_inHg input; Air_lb_hr output
function Air_lb_hr  = Calc_Air_Flow(Tatm_K,Pman_inHg,throttle,Patm_inHg)
%% Conversion Factors
inHg_to_Pa = 3386.39;
in2_to_m2 = 0.00064516;
kg_to_lb = 2.20462;
%% Constants
gamma = 1.4;
R = 287;
AirflowScaler = 0.69 * 0.95;
DischargeCoeff = 0.6;
th = 70*throttle;
D = 2.75;

Patm_Pa = Patm_inHg * inHg_to_Pa;
Pman_Pa = Pman_inHg * inHg_to_Pa;
A_in2 = (pi/4) * D^2 *  (0.01 + (1-0.01)*(1 - cosd(th)));
A_m2 = A_in2 * in2_to_m2;

Threshold_X = (2/(gamma+1))^(gamma/(gamma-1));

x = Threshold_X;

MAF = sqrt((2*gamma/(gamma-1))*(x^(2/gamma)-x^((gamma+1)/gamma)));

MassFlux_kgm2s = MAF*Patm_Pa/sqrt(R*Tatm_K);
MassFlow_kgs = MassFlux_kgm2s * A_m2; 

Air_lb_hr = AirflowScaler*DischargeCoeff*MassFlow_kgs*3600*kg_to_lb;
end

== matlab function DA40_Flight_Model/Stochastic Model/Navigation1/Flight Mechanics and Systems Models/Engine + Prop Model/Subsystem/Engine Shaft Power and Torque Model ==
  data: wdot_f input; PF input; BSFC input; P_shaft output
function P_shaft  = fcn(wdot_f,PF,BSFC)

P_shaft = PF*wdot_f/BSFC; %hp

% Q_drive = P_shaft*746/Omega; %Nm


end

== matlab function DA40_Flight_Model/Stochastic Model/Navigation1/Flight Mechanics and Systems Models/Engine + Prop Model/Subsystem/MATLAB Function ==
  data: X input; Aircraft_Airspeed output
function Aircraft_Airspeed = Calc_AC_Speed(X)
phi = X(10);
theta = X(11);
ps = X(12);

C_n_b = [1 0 0;0 cos(phi) sin(phi); 0 -sin(phi) cos(phi)]*...
    [cos(theta) 0 -sin(theta); 0 1 0; sin(theta) 0 cos(theta)]*...
    [cos(ps) sin(ps) 0; -sin(ps) cos(ps) 0; 0 0 1];

Aircraft_Airspeed = norm(C_n_b*(X(1:3)));
end

== matlab function DA40_Flight_Model/Stochastic Model/Navigation1/Flight Mechanics and Systems Models/Engine + Prop Model/Subsystem/Manifold Pressure Calculation ==
  data: throttle input; Patm_inHg input; N input; Pman_inHg output; throttle output; Patm_inHg output
function [Pman_inHg,throttle,Patm_inHg]  = fcn(throttle,Patm_inHg,N)

Pman_inHg = Patm_inHg + (0.007*throttle - 0.0086)*N;

end

== matlab function DA40_Flight_Model/Stochastic Model/Navigation1/Flight Mechanics and Systems Models/Engine + Prop Model/Subsystem/Propeller Dynamics ==
  data: V input; power input; Q_drive input size=1; Prop_Pitch input; rho input; n input; T output; Q output; eta_p output size=1; dOmega_dt output
function [T,Q,eta_p,dOmega_dt] = VarP_PropDynamics(V,power, Q_drive,Prop_Pitch,rho,n)

T = 0;
Q = 0;
eta_p = 0;
dOmega_dt = 0;

coder.extrinsic('griddedInterpolant')
coder.extrinsic('CTCQPropeff')

[T,Q,eta_p,dOmega_dt] = CTCQPropeff(Prop_Pitch,power,Q_drive,rho,V,n,[]);

end

== matlab function DA40_Flight_Model/Stochastic Model/Navigation1/Flight Mechanics and Systems Models/Gravity/MATLAB Function ==
  data: X input; F_grav_b output; Mass_Properties input; CG input; M_grav_b output
function [F_grav_b,M_grav_b] = Grav_Forces(X,Mass_Properties,CG)
%% Defining State Vector to Code Easier
u = X(1);
v = X(2);
w = X(3);
p = X(4);
q = X(5);
r = X(6);
x = X(7);
y = X(8);
z = X(9);
phi = X(10);
theta = X(11);
psi = X(12);

g = 9.81;

F_grav_b = Mass_Properties.*[-g*sin(theta);g*sin(phi)*cos(theta);g*cos(phi)*cos(theta)];

M_grav_b = cross(CG,F_grav_b);

== matlab function DA40_Flight_Model/Truth Model/Navigation1/Flight Mechanics and Systems Models/Engine + Prop Model/Subsystem/Air Flow Rate Exam 1 ==
  data: Tatm_K input; Pman_inHg input; throttle input; Patm_inHg input; Air_lb_hr output
function Air_lb_hr  = Calc_Air_Flow(Tatm_K,Pman_inHg,throttle,Patm_inHg)
%% Conversion Factors
inHg_to_Pa = 3386.39;
in2_to_m2 = 0.00064516;
kg_to_lb = 2.20462;
%% Constants
gamma = 1.4;
R = 287;
AirflowScaler = 0.69 * 0.95;
DischargeCoeff = 0.6;
th = 70*throttle;
D = 2.75;

Patm_Pa = Patm_inHg * inHg_to_Pa;
Pman_Pa = Pman_inHg * inHg_to_Pa;
A_in2 = (pi/4) * D^2 *  (0.01 + (1-0.01)*(1 - cosd(th)));
A_m2 = A_in2 * in2_to_m2;

Threshold_X = (2/(gamma+1))^(gamma/(gamma-1));

x = Threshold_X;

MAF = sqrt((2*gamma/(gamma-1))*(x^(2/gamma)-x^((gamma+1)/gamma)));

MassFlux_kgm2s = MAF*Patm_Pa/sqrt(R*Tatm_K);
MassFlow_kgs = MassFlux_kgm2s * A_m2; 

Air_lb_hr = AirflowScaler*DischargeCoeff*MassFlow_kgs*3600*kg_to_lb;
end

== matlab function DA40_Flight_Model/Truth Model/Navigation1/Flight Mechanics and Systems Models/Engine + Prop Model/Subsystem/Engine Shaft Power and Torque Model ==
  data: wdot_f input; PF input; BSFC input; P_shaft output
function P_shaft  = fcn(wdot_f,PF,BSFC)

P_shaft = PF*wdot_f/BSFC; %hp

% Q_drive = P_shaft*746/Omega; %Nm


end

== matlab function DA40_Flight_Model/Truth Model/Navigation1/Flight Mechanics and Systems Models/Engine + Prop Model/Subsystem/MATLAB Function ==
  data: X input; Aircraft_Airspeed output
function Aircraft_Airspeed = Calc_AC_Speed(X)
phi = X(10);
theta = X(11);
ps = X(12);

C_n_b = [1 0 0;0 cos(phi) sin(phi); 0 -sin(phi) cos(phi)]*...
    [cos(theta) 0 -sin(theta); 0 1 0; sin(theta) 0 cos(theta)]*...
    [cos(ps) sin(ps) 0; -sin(ps) cos(ps) 0; 0 0 1];

Aircraft_Airspeed = norm(C_n_b*(X(1:3)));
end

== matlab function DA40_Flight_Model/Truth Model/Navigation1/Flight Mechanics and Systems Models/Engine + Prop Model/Subsystem/Manifold Pressure Calculation ==
  data: throttle input; Patm_inHg input; N input; Pman_inHg output; throttle output; Patm_inHg output
function [Pman_inHg,throttle,Patm_inHg]  = fcn(throttle,Patm_inHg,N)

Pman_inHg = Patm_inHg + (0.007*throttle - 0.0086)*N;

end

== matlab function DA40_Flight_Model/Truth Model/Navigation1/Flight Mechanics and Systems Models/Engine + Prop Model/Subsystem/Propeller Dynamics ==
  data: V input; power input; Q_drive input size=1; Prop_Pitch input; rho input; n input; T output; Q output; eta_p output size=1; dOmega_dt output
function [T,Q,eta_p,dOmega_dt] = VarP_PropDynamics(V,power, Q_drive,Prop_Pitch,rho,n)

T = 0;
Q = 0;
eta_p = 0;
dOmega_dt = 0;

coder.extrinsic('griddedInterpolant')
coder.extrinsic('CTCQPropeff')

[T,Q,eta_p,dOmega_dt] = CTCQPropeff(Prop_Pitch,power,Q_drive,rho,V,n,[]);

end

== matlab function DA40_Flight_Model/Stochastic Model/Navigation1/Flight Mechanics and Systems Models/Strip Theory Aero + Propulsive Forces/Strip_Theory_Modeling ==
  data: atmos input; X input; U input; stripGeom input; Strip_Theory_Forces output; Strip_Theory_Moments output
function [Strip_Theory_Forces,Strip_Theory_Moments] = Strip_Theory(atmos,X,U,stripGeom)
Strip_Theory_Forces = [0;0;0];
Strip_Theory_Moments = [0;0;0];

coder.extrinsic('griddedInterpolant')
coder.extrinsic('AC_Strip_Theory')

[Strip_Theory_Forces,Strip_Theory_Moments] = AC_Strip_Theory(atmos(4),X,U,stripGeom);

== matlab function DA40_Flight_Model/Truth Model/Navigation1/Flight Mechanics and Systems Models/Gravity/MATLAB Function ==
  data: X input; F_grav_b output; Mass_Properties input; CG input; M_grav_b output
function [F_grav_b,M_grav_b] = Grav_Forces(X,Mass_Properties,CG)
%% Defining State Vector to Code Easier
u = X(1);
v = X(2);
w = X(3);
p = X(4);
q = X(5);
r = X(6);
x = X(7);
y = X(8);
z = X(9);
phi = X(10);
theta = X(11);
psi = X(12);

g = 9.81;

F_grav_b = Mass_Properties.*[-g*sin(theta);g*sin(phi)*cos(theta);g*cos(phi)*cos(theta)];

M_grav_b = cross(CG,F_grav_b);

== matlab function DA40_Flight_Model/Truth Model/Navigation1/Flight Mechanics and Systems Models/Strip Theory Aero + Propulsive Forces/Strip_Theory_Modeling ==
  data: atmos input; X input; U input; stripGeom input; Strip_Theory_Forces output; Strip_Theory_Moments output
function [Strip_Theory_Forces,Strip_Theory_Moments] = Strip_Theory(atmos,X,U,stripGeom)
Strip_Theory_Forces = [0;0;0];
Strip_Theory_Moments = [0;0;0];

coder.extrinsic('griddedInterpolant')
coder.extrinsic('AC_Strip_Theory')

[Strip_Theory_Forces,Strip_Theory_Moments] = AC_Strip_Theory(atmos(4),X,U,stripGeom);

== matlab function DA40_Flight_Model/Truth Model/Control/Subsystem3/MATLAB Function ==
  data: X input; Aircraft_Airspeed output
function Aircraft_Airspeed = Calc_AC_Speed(X)
Aircraft_Airspeed = norm(X(1:3));
end

== matlab function DA40_Flight_Model/MATLAB Function ==
  settings: updateMethod=DISCRETE  sampleTime=Time_Step
  data: M_ib_b input; F_ib_b input; predictedStates input size=14; trueF_ib_b input; trueM_ib_b input; estimatedStates output size=14; truereceiverStates output; varCarr output; varPsr output; resCarr output; resPsr output; receiverStates input; time input; rinexFilePath input; predictedCovariance input; estimatedCovariance output; year parameter; month parameter; day parameter; oldCN0 input; oldAmplitude input; oldNoise input; newCN0 output; newAmplitude output; newNoise output; newPhase output; oldPhase input; initCN0 parameter; Time_Step parameter; svStates output; clkVar parameter; variance parameter; Q parameter
function [estimatedStates,truereceiverStates, varCarr, varPsr, resCarr, resPsr,estimatedCovariance,newCN0,newAmplitude,newNoise,newPhase,svStates] = ...
    VectorTracking(M_ib_b,F_ib_b,predictedStates,trueF_ib_b,trueM_ib_b,receiverStates,time,rinexFilePath,predictedCovariance, year,month, day,oldCN0,oldAmplitude,oldNoise...
    ,oldPhase,initCN0,Time_Step,clkVar, variance,Q)

truereceiverStates = zeros(14,1);
estimatedStates = zeros(14,1);
estimatedCovariance = zeros(14);
resPsr = zeros(1,31);
resCarr = zeros(1,31);
varPsr = zeros(1,31);
varCarr = zeros(1,31);
newCN0 = zeros(1,31);
newAmplitude = zeros(1,31);
newNoise = zeros(1,31);
newPhase = zeros(1,31);
svStates = zeros(7,31);

coder.extrinsic("VectorTracking")
coder.extrinsic("flat2ecef")
coder.extrinsic("ecef2flat")
coder.extrinsic("genSatelliteStates")
coder.extrinsic("calcPsr")
coder.extrinsic("genCorrelatorResiduals")
coder.extrinsic("calcErrors")
coder.extrinsic("calcCodeError")
coder.extrinsic("calcCorrelators")
coder.extrinsic("calcFLLError")
coder.extrinsic("calcDLLError")
coder.extrinsic("calcPsrRes")
coder.extrinsic("calcCarrRes")
coder.extrinsic("calcResVariances")
coder.extrinsic("calculateCovariance")
coder.extrinsic("formZ")
coder.extrinsic("formH")
coder.extrinsic("formR")
coder.extrinsic("calcL")
coder.extrinsic("updateState")
coder.extrinsic("updateCovariance")

[estimatedStates,truereceiverStates,resPsr,resCarr,varPsr,varCarr,estimatedCovariance,newCN0,newAmplitude,newNoise,newPhase,svStates] = ...
    VectorTracking(F_ib_b,M_ib_b,predictedStates,trueF_ib_b,trueM_ib_b,receiverStates,predictedCovariance,rinexFilePath,time,year,month,day,oldCN0,oldAmplitude,...
    oldNoise,oldPhase,initCN0,Time_Step,variance,clkVar,Q);

stop = 1;

end

== matlab function DA40_Flight_Model/Truth Model/Environment/MATLAB Function7 ==
  data: RotAngles input; DCM output; RotSequence input
function DCM = MyDCMFunction(RotAngles,RotSequence)
n = length(RotSequence);
Matrix = zeros(3,3,3);
for i = 1:n
    k = RotSequence(i);
    switch k
        case 1
            Matrix(:,:,i) = [1 0 0;0 cosd(RotAngles(i)) -sind(RotAngles(i));0 sind(RotAngles(i)) cosd(RotAngles(i))];
        case 2
            Matrix(:,:,i) = [cosd(RotAngles(i)) 0 sind(RotAngles(i));0 1 0;-sind(RotAngles(i)) 0 cosd(RotAngles(i))];
        case 3
            Matrix(:,:,i) = [cosd(RotAngles(i)) -sind(RotAngles(i)) 0;sind(RotAngles(i)) cosd(RotAngles(i)) 0;0 0 1];
    end
end
p = 1;
while p < n
    Matrix(:,:,p+1) = Matrix(:,:,p) * Matrix(:,:,p+1);
    p = p + 1;
end
DCM = Matrix(:,:,p);
end
